simulink model "PubIfDecisionTOS_MDL"  (R2020b)
settings: configuration reference "DspaceConfig" (kept outside this file)
PostLoadFcn:
  | if any(exist('dsrtsu_mdlpostloadfcn', 'file') ~= 0), dsrtsu_mdlpostloadfcn('Execute', bdroot); end
InitFcn:
  | , if any(exist('dsmpb_private', 'file') ~= 0), dsmpb_private('dsmpb_mdlclblib', 'Init', bdroot); end,
undefined symbols (not defined in the file or in its folder): C_TOS_ACCEgoRAxletoFbumplength_m, C_TOS_ACCTargetFront_Flag, C_TOS_AEBJAPedObjDxThre_Val, C_TOS_AEBJAPedObjDyThre_Val, C_TOS_AEBJATargetSize_Val, C_TOS_AEBJAVehObjDxThre_Val, C_TOS_AEBJAVehObjDyThre_Val, C_TOS_AEBJuncPedTargetSize_Val, C_TOS_AEBLatObjDxThre_Val, C_TOS_AEBLatPedDyThre_Val, C_TOS_AEBLatTargetSize_Val, C_TOS_AEBLongTargetInEgoFront_Flag, C_TOS_axAbsGround_Parameter, C_TOS_CameraConfirmedFlag, C_TOS_CNsubjWidth, C_TOS_CurrentLaneCoreMinWidth_Val, C_TOS_CutInProb_Val_Zero, C_TOS_CutOutProb_Val_Zero, C_TOS_D2R_Val, C_TOS_DefaultValueObjectToCenterLine_dy, C_TOS_EgoCarWidth_Val, C_TOS_EgoDxRefPoint_m, C_TOS_EgoRAxletoFbumplength_m, C_TOS_HalfWidthVehicle_Con, C_TOS_HWA_CurrentLaneFlag, C_TOS_HWA_LeftLaneFlag, C_TOS_HWA_MovingDir_Vaild, C_TOS_HWA_MovState_Vaild, C_TOS_HWA_RightLaneFlag, C_TOS_LaneLineCourseErrorFront, C_TOS_LaneLineCourseErrorRear, C_TOS_MotorbikeDefaultWidth_m, C_TOS_NumberOfEffectiveTargets, C_TOS_Obj_Age_Val, C_TOS_Objdx_Constraint_Val, C_TOS_ObjectDefaultWidth_m, C_TOS_ObjInCurrentLane_Val, C_TOS_ObjInCurrentLaneValid, C_TOS_ObjInLeftLaneValid, C_TOS_ObjInRightLaneValid, C_TOS_ObjNotInCurrentLane_Val, C_TOS_ObjNotREElementType, C_TOS_ObjPredictDis_dy_ConstantVal_Zeros, C_TOS_ObjToCenterLine_ConstantVal_Zeros, C_TOS_OFMObjIDInvilad_Val, C_TOS_PIL_LatDisCons_Val_zero, C_TOS_PIL_ObjectCutInFlag_b, C_TOS_PIL_ObjectCutOutFlag_b, C_TOS_PIL_ObjLaneProb_al_Val, C_TOS_PP_ObjFusType_FC_Confirm_b, C_TOS_PP_ObjFusType_FC_FR_Confirm_b, C_TOS_PP_ObjFusType_FR_Confirm_b, C_TOS_RE_80BoolDefault_Val, C_TOS_RE_80Single181Default_Val, C_TOS_RE_80Single255Default_Val, C_TOS_RE_80Uint8Default_Val, C_TOS_RE_D2R, C_TOS_RE_D_180_Val, C_TOS_RE_InvalidObjectID_Val, C_TOS_RE_InvalidTargetChainDir_Val ... (+142)
libraries: simulink x1650, TOS_LIB x361, canfdmsglib x14
(part 39 of 69)

== system PubIfDecisionTOS_MDL/TOS_20201112/TOS_2012080320/TOS/AEB/TOS_AEBLong/AEBLong_Confirm/AEBLong/AEBLong_TrgConfirm/AEBLongTrgJudg ==
  ObjectID : Inport
  Object_DX : Inport  Port=2
  Object_ObstacleProb : Inport  Port=3
  Object_ExistProb : Inport  Port=4
  Object_Fus_Type : Inport  Port=5
  object_MovingState : Inport  Port=6
  Object_HeadingAngle : Inport  Port=7
  Object_Type : Inport  Port=8
  VIE_EgoVelocity : Inport  Port=9
  PIL_LeftLaneProb : Inport  Port=10
  PIL_CurrentLaneProb : Inport  Port=11
  PIL_RightLaneProb : Inport  Port=12
  PP_MovingStateSignalProcessing : Inport  Port=13
  PP_ObjMovingDirSignalProcessing : Inport  Port=14
  PP_ObjectToCenterLine_dy : Inport  Port=15
  PP_CurrentLaneWidth : Inport  Port=16
  TLJ_TargetInCLValidityflg : Inport  Port=17
  Object_DY : Inport  Port=18
  PP_ObjFusType_FC_FR_Confirm : Inport  Port=19
  PP_ObjFusType_FR_Confirm : Inport  Port=20
  PP_ObjFusType_FC_Confirm : Inport  Port=21
  Object_VX : Inport  Port=22
  Object_VY : Inport  Port=23
  PIL_OverlapRatio : Inport  Port=24
  AEBLong_Target_ID_K1 : Inport  Port=25
  AEBLong_Target_ID_K2 : Inport  Port=26
  AEBLong_Target_MovState_K1 : Inport  Port=27
  AEBLong_Target_MovState_K2 : Inport  Port=28
  SteerWheelAng : Inport  Port=29
  SteerWheelSpd : Inport  Port=30
  AEBLong_OverlapRatio : Subsystem
  Bus Creator : BusCreator  Inputs=30
  Bus Selector : BusSelector  OutputSignals=object_MovingState,PP_ObjFusType_FC_FR_Confirm,PP_ObjFusType_FR_Confirm,AEBLong_Target_ID_K1,AEBLong_Target_ID_K2,AEBLong_Target_MovState_K1,AEBLong_Target_MovState_K2,ObjectID
  Bus Selector1 : BusSelector  OutputSignals=object_MovingState,PP_ObjMovingDirSignalProcessing,Object_HeadingAngle,Object_VX,Object_VY,VIE_EgoVelocity,SteerWheelAng,AEBLong_Target_ID_K1,AEBLong_Target_ID_K2,AEBLong_Target_MovState_K1,AEBLong_Target_MovState_K2,ObjectID
  Bus Selector2 : BusSelector  OutputSignals=Object_DX,TLJ_TargetInCLValidityflg
  Bus Selector3 : BusSelector  OutputSignals=VIE_EgoVelocity,Object_DX
  Bus Selector4 : BusSelector  OutputSignals=Object_ExistProb
  Bus Selector5 : BusSelector  OutputSignals=PP_ObjFusType_FR_Confirm,object_MovingState,Object_DX,PP_ObjectToCenterLine_dy,Object_Type
  Bus Selector6 : BusSelector  OutputSignals=Object_DY,Object_DX,Object_Type
  Bus Selector7 : BusSelector  OutputSignals=Object_ObstacleProb,AEBLong_Target_ID_K1,ObjectID
  Bus Selector8 : BusSelector  OutputSignals=SteerWheelAng,SteerWheelSpd
  Bus Selector9 : BusSelector  OutputSignals=PIL_OverlapRatio
  Constant : Constant  OutDataTypeStr=boolean
  Constant2 : Constant  OutDataTypeStr=boolean
  Logical Operator : Logic  Inputs=10  AllPortsSameDT=off  OutDataTypeStr=boolean
  TOS_AEBLong_Dy : Subsystem
  TOS_AEBLong_ObjFusType : Subsystem
  TOS_AEBLong_ObstacleProb : Subsystem
  TOS_AEBLong_SteerWheelAngConfirm : Subsystem
  TOS_AEBLong_TargetDis : Subsystem
  TOS_AEBLong_TargetExistProb : Subsystem
  TOS_AEBLong_TargetInEgoFront : Subsystem
  TOS_AEBLong_TargetMovingDir : Subsystem
  TOS_AEB_Stockade : Subsystem
  Terminator : Terminator
  Terminator1 : Terminator
  TOS_AEBLong_TargetConditionJudge : Outport
  TOS_AEBLong_TargetDis_ObserVale : Outport  Port=2
  TOS_AEBLong_ObstacleProb_ObserVale : Outport  Port=3
  TOS_AEBLong_TargetExistProb_ObserVale : Outport  Port=4
  TOS_AEBLong_ObjFusType_ObserVale : Outport  Port=5
  TOS_AEBLong_TargetInEgoFront_ObserVale : Outport  Port=6
  TOS_AEBLong_TargetMovingDir_ObserVale : Outport  Port=7
  TOS_AEB_Stockade_ObserVale : Outport  Port=8
  TOS_AEBLong_TargetDy_ObserVale : Outport  Port=9
  TOS_AEBLong_SteerWheelAngConfirm_ObserVale : Outport  Port=10
  TOS_AEBLong_OverlapRatio_ObserVale : Outport  Port=11
  wires:
  TOS_AEBLong_ObjFusType/1(TOS_AEBLongAEBLongObjFusType) -> [TOS_AEBLong_ObjFusType_ObserVale], Logical Operator/4  "TOS_AEBLong_ObjFusType"
  TOS_AEBLong_ObstacleProb/1(TOS_AEBLongObstacleProbFlag) -> Logical Operator/2, [TOS_AEBLong_ObstacleProb_ObserVale]  "TOS_AEBLong_ObstacleProb"
  TOS_AEBLong_TargetExistProb/1(TOS_AEBLongTargetExistProbFlag) -> [TOS_AEBLong_TargetExistProb_ObserVale], Logical Operator/3  "TOS_AEBLong_TargetExistProb"
  Constant2/1 -> [TOS_AEB_Stockade_ObserVale], Logical Operator/7  "TOS_AEB_Stockade"
  TOS_AEBLong_TargetMovingDir/1(TOS_AEBLongMovingDirFlg) -> [TOS_AEBLong_TargetMovingDir_ObserVale], Logical Operator/6  "TOS_AEBLong_TargetMovingDir"
  TOS_AEBLong_TargetInEgoFront/1(TOS_TargetInEgoFrontflg) -> [TOS_AEBLong_TargetInEgoFront_ObserVale], Logical Operator/5  "TOS_AEBLong_TargetInEgoFront"
  TOS_AEBLong_TargetDis/1(TOS_TargetDxThreflg) -> Logical Operator/1, [TOS_AEBLong_TargetDis_ObserVale]  "TOS_AEBLong_TargetDis"
  Object_Fus_Type/1 -> Bus Creator/5  "Object_Fus_Type"
  PP_ObjMovingDirSignalProcessing/1 -> Bus Creator/14  "PP_ObjMovingDirSignalProcessing"
  PP_ObjectToCenterLine_dy/1 -> Bus Creator/15  "PP_ObjectToCenterLine_dy"
  VIE_EgoVelocity/1 -> Bus Creator/9  "VIE_EgoVelocity"
  Object_ExistProb/1 -> Bus Creator/4  "Object_ExistProb"
  PIL_CurrentLaneProb/1 -> Bus Creator/11  "PIL_CurrentLaneProb"
  PP_MovingStateSignalProcessing/1 -> Bus Creator/13  "PP_MovingStateSignalProcessing"
  PIL_RightLaneProb/1 -> Bus Creator/12  "PIL_RightLaneProb"
  PIL_LeftLaneProb/1 -> Bus Creator/10  "PIL_LeftLaneProb"
  Object_ObstacleProb/1 -> Bus Creator/3  "Object_ObstacleProb"
  Object_DX/1 -> Bus Creator/2  "Object_DX"
  PP_CurrentLaneWidth/1 -> Bus Creator/16  "PP_CurrentLaneWidth"
  Bus Selector1/2 -> TOS_AEBLong_TargetMovingDir/2(PP_ObjMovingDirSignalProcessing)  "<PP_ObjMovingDirSignalProcessing>"
  Bus Selector2/1 -> TOS_AEBLong_TargetInEgoFront/1(Object_Dx)  "<Object_DX>"
  Bus Selector7/1 -> TOS_AEBLong_ObstacleProb/1(Object_ObstacleProb)  "<Object_ObstacleProb>"
  Bus Selector3/1 -> TOS_AEBLong_TargetDis/1(VIE_EgoVelocity)  "<VIE_EgoVelocity>"
  Bus Selector4/1 -> TOS_AEBLong_TargetExistProb/1(Object_ExistProb)  "<Object_ExistProb>"
  Bus Selector3/2 -> TOS_AEBLong_TargetDis/2(Object_Dx)  "<Object_DX>"
  TLJ_TargetInCLValidityflg/1 -> Bus Creator/17  "TLJ_TargetInCLValidityflg"
  Bus Selector2/2 -> TOS_AEBLong_TargetInEgoFront/2(TLJ_TargetInCLValidityflg)  "<TLJ_TargetInCLValidityflg>"
  Bus Selector5/1 -> TOS_AEB_Stockade/1(PP_ObjFusType_FR_Confirm)  "<PP_ObjFusType_FR_Confirm>"
  Bus Selector5/2 -> TOS_AEB_Stockade/2(object_MovingState)  "<object_MovingState>"
  Bus Selector5/3 -> TOS_AEB_Stockade/3(Object_DX)  "<Object_DX>"
  Bus Selector5/4 -> TOS_AEB_Stockade/4(ObjectToCenterLine_dy)  "<PP_ObjectToCenterLine_dy>"
  [TOS_AEBLong_TargetDis_ObserVale] -> TOS_AEBLong_TargetDis_ObserVale/1
  [TOS_AEBLong_ObstacleProb_ObserVale] -> TOS_AEBLong_ObstacleProb_ObserVale/1
  [TOS_AEBLong_ObjFusType_ObserVale] -> TOS_AEBLong_ObjFusType_ObserVale/1
  [TOS_AEBLong_TargetExistProb_ObserVale] -> TOS_AEBLong_TargetExistProb_ObserVale/1
  [TOS_AEBLong_TargetInEgoFront_ObserVale] -> TOS_AEBLong_TargetInEgoFront_ObserVale/1
  [TOS_AEBLong_TargetMovingDir_ObserVale] -> TOS_AEBLong_TargetMovingDir_ObserVale/1
  [TOS_AEB_Stockade_ObserVale] -> TOS_AEB_Stockade_ObserVale/1
  TOS_AEBLong_Dy/1(TOS_AEBLongDy) -> [TOS_AEBLong_TargetDy_ObserVale], Logical Operator/8  "TOS_AEBLongDyFlag"
  Object_DY/1 -> Bus Creator/18  "Object_DY"
  [TOS_AEBLong_TargetDy_ObserVale] -> TOS_AEBLong_TargetDy_ObserVale/1
  object_MovingState/1 -> Bus Creator/6  "object_MovingState"
  Bus Selector/1 -> TOS_AEBLong_ObjFusType/1(object_MovingState)  "<object_MovingState>"
  Object_HeadingAngle/1 -> Bus Creator/7  "Object_HeadingAngle"
  Bus Selector1/3 -> TOS_AEBLong_TargetMovingDir/3(Object_HeadingAngle)  "<Object_HeadingAngle>"
  Object_Type/1 -> Bus Creator/8  "Object_Type"
  Bus Selector5/5 -> TOS_AEB_Stockade/5(Object_Type)  "<Object_Type>"
  Bus Selector1/1 -> TOS_AEBLong_TargetMovingDir/1(object_MovingState)  "<object_MovingState>"
  SteerWheelSpd/1 -> Bus Creator/20  "SteerWheelSpd"
  SteerWheelAng/1 -> Bus Creator/19  "SteerWheelAng"
  Bus Selector8/1 -> TOS_AEBLong_SteerWheelAngConfirm/1(SteerWheelAng)  "<SteerWheelAng>"
  Bus Selector8/2 -> TOS_AEBLong_SteerWheelAngConfirm/2(SteerWheelSpd)  "<SteerWheelSpd>"
  [TOS_AEBLong_SteerWheelAngConfirm_ObserVale] -> TOS_AEBLong_SteerWheelAngConfirm_ObserVale/1
  TOS_AEBLong_SteerWheelAngConfirm/1(TOS_AEBLong_SteerWheelAngConfirm) -> Logical Operator/9, [TOS_AEBLong_SteerWheelAngConfirm_ObserVale]  "TOS_AEBLong_SteerWheelAngConfirm"
  ObjectID/1 -> Bus Creator/1  "ObjectID"
  Logical Operator/1 -> TOS_AEBLong_TargetConditionJudge/1
  PP_ObjFusType_FC_FR_Confirm/1 -> Bus Creator/21  "PP_ObjFusType_FC_FR_Confirm"
  PP_ObjFusType_FR_Confirm/1 -> Bus Creator/22  "PP_ObjFusType_FR_Confirm"
  PP_ObjFusType_FC_Confirm/1 -> Bus Creator/23  "PP_ObjFusType_FC_Confirm"
  Bus Selector/2 -> TOS_AEBLong_ObjFusType/2(PP_ObjFusType_FC_FR_Confirm)  "<PP_ObjFusType_FC_FR_Confirm>"
  Bus Selector/3 -> TOS_AEBLong_ObjFusType/3(PP_ObjFusType_FR_Confirm)  "<PP_ObjFusType_FR_Confirm>"
  Bus Creator/1 -> Bus Selector6/1, Bus Selector9/1, Bus Selector8/1, Bus Selector5/1, Bus Selector1/1, Bus Selector2/1, Bus Selector/1, Bus Selector4/1, Bus Selector7/1, Bus Selector3/1
  Bus Selector6/2 -> TOS_AEBLong_Dy/2(Object_DX)  "<Object_DX>"
  Bus Selector6/1 -> TOS_AEBLong_Dy/1(Object_DY)  "<Object_DY>"
  Bus Selector6/3 -> TOS_AEBLong_Dy/3(<Object_Type>)  "<Object_Type>"
  Object_VY/1 -> Bus Creator/25  "Object_VY"
  Object_VX/1 -> Bus Creator/24  "Object_VX"
  Bus Selector1/4 -> TOS_AEBLong_TargetMovingDir/4(Object_VX)  "<Object_VX>"
  Bus Selector1/5 -> TOS_AEBLong_TargetMovingDir/5(Object_VY)  "<Object_VY>"
  Bus Selector1/6 -> TOS_AEBLong_TargetMovingDir/6(VIE_EgoVelocity)  "<VIE_EgoVelocity>"
  Bus Selector1/7 -> TOS_AEBLong_TargetMovingDir/7(SteerWheelAngle)  "<SteerWheelAng>"
  PIL_OverlapRatio/1 -> Bus Creator/26  "PIL_OverlapRatio"
  Bus Selector9/1 -> AEBLong_OverlapRatio/1(PIL_OverlapRatio)  "<PIL_OverlapRatio>"
  Constant/1 -> [TOS_AEBLong_OverlapRatio_ObserVale], Logical Operator/10
  [TOS_AEBLong_OverlapRatio_ObserVale] -> TOS_AEBLong_OverlapRatio_ObserVale/1
  AEBLong_OverlapRatio/1(AEBLong_OverlapRatioFlag) -> Terminator/1
  TOS_AEB_Stockade/1(TOS_AEB_Stockade) -> Terminator1/1
  AEBLong_Target_ID_K1/1 -> Bus Creator/27  "AEBLong_Target_ID_K1"
  AEBLong_Target_ID_K2/1 -> Bus Creator/28  "AEBLong_Target_ID_K2"
  AEBLong_Target_MovState_K1/1 -> Bus Creator/29  "AEBLong_Target_MovState_K1"
  AEBLong_Target_MovState_K2/1 -> Bus Creator/30  "AEBLong_Target_MovState_K2"
  Bus Selector/4 -> TOS_AEBLong_ObjFusType/4(AEBLong_Target_ID_K1)  "<AEBLong_Target_ID_K1>"
  Bus Selector/5 -> TOS_AEBLong_ObjFusType/5(AEBLong_Target_ID_K2)  "<AEBLong_Target_ID_K2>"
  Bus Selector/6 -> TOS_AEBLong_ObjFusType/6(AEBLong_Target_MovState_K1)  "<AEBLong_Target_MovState_K1>"
  Bus Selector/7 -> TOS_AEBLong_ObjFusType/7(AEBLong_Target_MovState_K2)  "<AEBLong_Target_MovState_K2>"
  Bus Selector/8 -> TOS_AEBLong_ObjFusType/8(ObjectID)  "<ObjectID>"
  Bus Selector7/2 -> TOS_AEBLong_ObstacleProb/2(AEBLong_Target_ID_K1)  "<AEBLong_Target_ID_K1>"
  Bus Selector7/3 -> TOS_AEBLong_ObstacleProb/3(ObjectID)  "<ObjectID>"
  Bus Selector1/8 -> TOS_AEBLong_TargetMovingDir/8(AEBLong_Target_ID_K1)  "<AEBLong_Target_ID_K1>"
  Bus Selector1/9 -> TOS_AEBLong_TargetMovingDir/9(AEBLong_Target_ID_K2)  "<AEBLong_Target_ID_K2>"
  Bus Selector1/10 -> TOS_AEBLong_TargetMovingDir/10(AEBLong_Target_MovState_K1)  "<AEBLong_Target_MovState_K1>"
  Bus Selector1/11 -> TOS_AEBLong_TargetMovingDir/11(AEBLong_Target_MovState_K2)  "<AEBLong_Target_MovState_K2>"
  Bus Selector1/12 -> TOS_AEBLong_TargetMovingDir/12(ObjectID)  "<ObjectID>"

== system PubIfDecisionTOS_MDL/TOS_20201112/TOS_2012080320/TOS/AEB/TOS_AEBLong/AEBLong_Confirm/AEBLong/AEBLong_TrgConfirm/Subsystem ==
  Dx1stNearestObjIndex : Inport
  Object_ID : Inport  Port=2
  Object_DX : Inport  Port=3
  Object_ObstacleProb : Inport  Port=4
  Object_ExistProb : Inport  Port=5
  Object_Fus_Type : Inport  Port=6
  object_MovingState : Inport  Port=7
  Object_HeadingAngle : Inport  Port=8
  Object_Type : Inport  Port=9
  VIE_EgoVelocity : Inport  Port=10
  PIL_LeftLaneProb : Inport  Port=11
  PIL_CurrentLaneProb : Inport  Port=12
  PIL_RightLaneProb : Inport  Port=13
  PP_MovingStateSignalProcessing : Inport  Port=14
  PP_ObjMovingDirSignalProcessing : Inport  Port=15
  PP_ObjectToCenterLine_dy : Inport  Port=16
  TLJ_TargetInCLValidityflg : Inport  Port=17
  PP_CurrentLaneWidth : Inport  Port=18
  Object_DY : Inport  Port=19
  PP_ObjFusType_FC_FR_Confirm : Inport  Port=20
  PP_ObjFusType_FR_Confirm : Inport  Port=21
  PP_ObjFusType_FC_Confirm : Inport  Port=22
  Object_VX : Inport  Port=23
  Object_VY : Inport  Port=24
  PIL_OverlapRatio : Inport  Port=25
  AEBLong_Target_ID_K1 : Inport  Port=26
  AEBLong_Target_ID_K2 : Inport  Port=27
  AEBLong_Target_MovState_K1 : Inport  Port=28
  AEBLong_Target_MovState_K2 : Inport  Port=29
  Selector{,1..21} (22 alike) : Selector  InputPortWidth=80  IndexOptions=Index vector (port)  Indices=[1 3]  OutputSizes=1
  ObjectID : Outport
  ObjectDX : Outport  Port=2
  ObjectObstacleProb : Outport  Port=3
  ObjectExistProb : Outport  Port=4
  ObjectFus_Type : Outport  Port=5
  objectMovingState : Outport  Port=6
  ObjectHeadingAngle : Outport  Port=7
  ObjectType : Outport  Port=8
  VIEEgoVelocity : Outport  Port=9
  PILLeftLaneProb : Outport  Port=10
  PILCurrentLaneProb : Outport  Port=11
  PILRightLaneProb : Outport  Port=12
  PPMovingStateSignalProcessing : Outport  Port=13
  PPObjMovingDirSignalProcessing : Outport  Port=14
  PPObjectToCenterLine_dy : Outport  Port=15
  PPCurrentLaneWidth : Outport  Port=16
  TLJTargetInCLValidityflg : Outport  Port=17
  ObjectDY : Outport  Port=18
  PP_ObjFusType_FC_FR_Confirm_ : Outport  Port=19
  PP_ObjFusType_FR_Confirm_ : Outport  Port=20
  PP_ObjFusType_FC_Confirm_ : Outport  Port=21
  ObjectVX : Outport  Port=22
  ObjectVY : Outport  Port=23
  PILOverlapRatio : Outport  Port=24
  AEBLongTarget_ID_K2 : Outport  Port=25
  AEBLongTarget_ID_K1 : Outport  Port=26
  AEBLongTarget_MovState_K2 : Outport  Port=27
  AEBLongTarget_MovState_K1 : Outport  Port=28
  wires:
  Object_ID/1 -> Selector/1
  Object_ObstacleProb/1 -> Selector2/1
  Object_DX/1 -> Selector1/1
  Selector/1 -> ObjectID/1  "Object_ID"
  Object_ExistProb/1 -> Selector3/1
  Object_DY/1 -> Selector16/1
  Object_Fus_Type/1 -> Selector4/1
  object_MovingState/1 -> Selector5/1
  Object_HeadingAngle/1 -> Selector6/1
  Object_Type/1 -> Selector7/1
  PIL_LeftLaneProb/1 -> Selector8/1
  PIL_CurrentLaneProb/1 -> Selector9/1
  PIL_RightLaneProb/1 -> Selector10/1
  PP_MovingStateSignalProcessing/1 -> Selector11/1
  PP_ObjMovingDirSignalProcessing/1 -> Selector12/1
  PP_ObjectToCenterLine_dy/1 -> Selector13/1
  TLJ_TargetInCLValidityflg/1 -> Selector15/1
  Selector1/1 -> ObjectDX/1  "Object_DX"
  Selector2/1 -> ObjectObstacleProb/1  "Object_ObstacleProb"
  Selector3/1 -> ObjectExistProb/1  "Object_ExistProb"
  Selector4/1 -> ObjectFus_Type/1  "Object_Fus_Type"
  Selector5/1 -> objectMovingState/1  "object_MovingState"
  Selector6/1 -> ObjectHeadingAngle/1  "Object_HeadingAngle"
  Selector7/1 -> ObjectType/1  "Object_Type"
  VIE_EgoVelocity/1 -> VIEEgoVelocity/1  "VIE_EgoVelocity"
  Selector8/1 -> PILLeftLaneProb/1  "PIL_LeftLaneProb"
  Selector9/1 -> PILCurrentLaneProb/1  "PIL_CurrentLaneProb"
  Selector10/1 -> PILRightLaneProb/1  "PIL_RightLaneProb"
  Selector11/1 -> PPMovingStateSignalProcessing/1  "PP_MovingStateSignalProcessing"
  Selector12/1 -> PPObjMovingDirSignalProcessing/1  "PP_ObjMovingDirSignalProcessing"
  Selector13/1 -> PPObjectToCenterLine_dy/1  "PP_ObjectToCenterLine_dy"
  PP_CurrentLaneWidth/1 -> PPCurrentLaneWidth/1  "PP_CurrentLaneWidth"
  Selector15/1 -> TLJTargetInCLValidityflg/1  "TLJ_TargetInCLValidityflg"
  Selector16/1 -> ObjectDY/1  "Object_DY"
  PP_ObjFusType_FC_FR_Confirm/1 -> Selector14/1
  PP_ObjFusType_FR_Confirm/1 -> Selector17/1
  PP_ObjFusType_FC_Confirm/1 -> Selector18/1
  Selector18/1 -> PP_ObjFusType_FC_Confirm_/1
  Selector17/1 -> PP_ObjFusType_FR_Confirm_/1
  Selector14/1 -> PP_ObjFusType_FC_FR_Confirm_/1
  Selector19/1 -> ObjectVX/1
  Object_VX/1 -> Selector19/1
  Selector20/1 -> ObjectVY/1
  Object_VY/1 -> Selector20/1
  PIL_OverlapRatio/1 -> Selector21/1
  Dx1stNearestObjIndex/1 -> Selector1/2, Selector2/2, Selector3/2, Selector4/2, Selector5/2, Selector6/2, Selector7/2, Selector8/2, Selector9/2, Selector10/2, Selector11/2, Selector12/2, Selector13/2, Selector21/2, Selector20/2, Selector19/2, Selector18/2, Selector17/2, Selector14/2, Selector16/2, Selector15/2, Selector/2
  Selector21/1 -> PILOverlapRatio/1
  AEBLong_Target_ID_K1/1 -> AEBLongTarget_ID_K1/1  "AEBLong_Target_ID_K1"
  AEBLong_Target_ID_K2/1 -> AEBLongTarget_ID_K2/1  "AEBLong_Target_ID_K2"
  AEBLong_Target_MovState_K1/1 -> AEBLongTarget_MovState_K1/1
  AEBLong_Target_MovState_K2/1 -> AEBLongTarget_MovState_K2/1

== system PubIfDecisionTOS_MDL/TOS_20201112/TOS_2012080320/TOS/AEB/TOS_AEBLong/AEBLong_Target_PreJudge/AEBLONG_Target_PreFilt/AEBLONG_TargetPreCondJudge/AEBLONGTarget_Fence ==
  FR_Confirm : Inport
  Obj_MovingState : Inport  Port=2
  Object_ObstacleProb : Inport  Port=3
  Object_DY : Inport  Port=4
  Chart : Stateflow chart  TreatAsAtomicUnit=on
  Data Type Conversion1 : DataTypeConversion  OutDataTypeStr=Enum: OFM_OBJ_MOVINGSTATE_E
  TOS_AEBLONG_Target_FenceFlag : Outport
  wires:
  Chart/1(ObjectisFence_Flag) -> TOS_AEBLONG_Target_FenceFlag/1
  Object_DY/1 -> Chart/4(Object_DY)
  FR_Confirm/1 -> Chart/1(FR_Confirm)
  Obj_MovingState/1 -> Data Type Conversion1/1
  Object_ObstacleProb/1 -> Chart/3(Object_ObstacleProb)
  Data Type Conversion1/1 -> Chart/2(Obj_MovingState)

== system PubIfDecisionTOS_MDL/TOS_20201112/TOS_2012080320/TOS/AEB/TOS_AEBLong/AEBLong_Target_PreJudge/AEBLONG_Target_PreFilt/AEBLONG_TargetPreCondJudge/AEBLONGTarget_FusionType ==
  PP_ObjFusType_FC_FR_Confirm : Inport
  PP_ObjFusType_FR_Confirm : Inport  Port=2
  Compare To Constant5 : simulink/Logic and Bit Operations/Compare To Constant  relop===  const=C_TOS_PP_ObjFusType_FC_FR_Confirm_b  OutDataTypeStr=boolean
      settings: AttributesFormatString=C_TOS_PP_ObjFusType_FC_FR_Confirm_b = 1
  Compare To Constant6 : simulink/Logic and Bit Operations/Compare To Constant  relop===  const=C_TOS_PP_ObjFusType_FR_Confirm_b  OutDataTypeStr=boolean
      settings: AttributesFormatString=C_TOS_PP_ObjFusType_FR_Confirm_b = 1
  Logical Operator : Logic  Operator=OR  AllPortsSameDT=off  OutDataTypeStr=boolean
  TOS_AEBLONG_Target_FusionTypeFlag : Outport
  wires:
  Logical Operator/1 -> TOS_AEBLONG_Target_FusionTypeFlag/1
  Compare To Constant6/1 -> Logical Operator/2
  PP_ObjFusType_FC_FR_Confirm/1 -> Compare To Constant5/1
  PP_ObjFusType_FR_Confirm/1 -> Compare To Constant6/1
  Compare To Constant5/1 -> Logical Operator/1

== system PubIfDecisionTOS_MDL/TOS_20201112/TOS_2012080320/TOS/AEB/TOS_AEBLong/AEBLong_Target_PreJudge/AEBLONG_Target_PreFilt/AEBLONG_TargetPreCondJudge/AEBLONGTarget_PassedbyTarget ==
  note: 目标分裂处理
  FR_Confirm : Inport
  Obj_MovingState : Inport  Port=2
  Obj_Dx : Inport  Port=3
  AEBLONG_TargetP0_ID_K1 : Inport  Port=4
  AEBLONG_TargetP0_Dx_K1 : Inport  Port=5
  Object_ID : Inport  Port=6
  Add : Sum
  Compare To Constant : simulink/Logic and Bit Operations/Compare To Constant  relop=~=  const=C_TOS_OFMObjIDInvilad_Val  OutDataTypeStr=boolean
      settings: AttributesFormatString=C_TOS_OFMObjIDInvilad_Val = 0
  Compare To Constant1 : simulink/Logic and Bit Operations/Compare To Constant  relop===  const=C_TOS_PP_ObjFusType_FR_Confirm_b  OutDataTypeStr=boolean
      settings: AttributesFormatString=C_TOS_PP_ObjFusType_FC_Confirm_b = 1
  Compare To Constant2 : simulink/Logic and Bit Operations/Compare To Constant  relop===  const=OFM_OBJ_MOVINGSTATE_E.UNKNOWN  OutDataTypeStr=boolean
      settings: AttributesFormatString=OFM_OBJ_MOVINGSTATE_E.MOVING = 2
  Compare To Constant3 : simulink/Logic and Bit Operations/Compare To Constant  relop===  const=OFM_OBJ_MOVINGSTATE_E.INVALID  OutDataTypeStr=boolean
      settings: AttributesFormatString=OFM_OBJ_MOVINGSTATE_E.MOVING = 2
  Compare To Constant4 : simulink/Logic and Bit Operations/Compare To Constant  relop===  const=OFM_OBJ_MOVINGSTATE_E.STATIONARY  OutDataTypeStr=boolean
      settings: AttributesFormatString=OFM_OBJ_MOVINGSTATE_E.MOVING = 2
  Constant : Constant  OutDataTypeStr=single
  Constant1 : Constant  Value=0  OutDataTypeStr=boolean
  Constant2 : Constant  Value=0  OutDataTypeStr=boolean
  Data Type Conversion1 : DataTypeConversion  OutDataTypeStr=Enum: OFM_OBJ_MOVINGSTATE_E
  Logical Operator : Logic  Operator=OR  Inputs=3  AllPortsSameDT=off  OutDataTypeStr=boolean
  Logical Operator1 : Logic  AllPortsSameDT=off  OutDataTypeStr=boolean
  Logical Operator2 : Logic  AllPortsSameDT=off  OutDataTypeStr=boolean
  Relational Operator : RelationalOperator  Operator=<  OutDataTypeStr=boolean  RndMeth=Simplest
  Relational Operator1 : RelationalOperator  Operator=~=  OutDataTypeStr=boolean  RndMeth=Simplest
  Switch : Switch  Criteria=u2 ~= 0
  Switch1 : Switch  Criteria=u2 ~= 0
  TOS_AEBLONG_Target_PassedbyTarget_Flag : Outport
  wires:
  Switch/1 -> TOS_AEBLONG_Target_PassedbyTarget_Flag/1
  Compare To Constant3/1 -> Logical Operator/1
  Compare To Constant/1 -> Logical Operator2/1
  Constant/1 -> Add/2
  Obj_MovingState/1 -> Data Type Conversion1/1
  Obj_Dx/1 -> Relational Operator/1
  Relational Operator/1 -> Switch1/1
  Compare To Constant1/1 -> Logical Operator1/1
  Compare To Constant2/1 -> Logical Operator/2
  FR_Confirm/1 -> Compare To Constant1/1
  Logical Operator1/1 -> Switch1/2
  Switch1/1 -> Switch/1
  Add/1 -> Relational Operator/2
  Logical Operator/1 -> Logical Operator1/2
  Constant2/1 -> Switch/3
  AEBLONG_TargetP0_Dx_K1/1 -> Add/1
  Constant1/1 -> Switch1/3
  Compare To Constant4/1 -> Logical Operator/3
  AEBLONG_TargetP0_ID_K1/1 -> Relational Operator1/1, Compare To Constant/1
  Data Type Conversion1/1 -> Compare To Constant4/1, Compare To Constant2/1, Compare To Constant3/1
  Object_ID/1 -> Relational Operator1/2
  Relational Operator1/1 -> Logical Operator2/2
  Logical Operator2/1 -> Switch/2

== system PubIfDecisionTOS_MDL/TOS_20201112/TOS_2012080320/TOS/AEB/TOS_AEBLong/AEBLong_Target_PreJudge/AEBLONG_Target_PreFilt/AEBLONG_TargetPreCondJudge/REElementType ==
  PP_REElementType : Inport
  Compare To Constant1 : simulink/Logic and Bit Operations/Compare To Constant  relop===  const=C_TOS_ObjNotREElementType  OutDataTypeStr=boolean
      settings: AttributesFormatString=%<const> = 0
  TOS_AEBLONG_Target_REElementType : Outport
  wires:
  Compare To Constant1/1 -> TOS_AEBLONG_Target_REElementType/1
  PP_REElementType/1 -> Compare To Constant1/1

== system PubIfDecisionTOS_MDL/TOS_20201112/TOS_2012080320/TOS/LC_LCKie_ELK/TOS_HWA/CurrentLane/HWA_CurrentLane_Target/HWA_CLF_Target_1/HWA_CLF_Target ==
  HWA_CLF_Target_1_Index : Inport
  Object_Fus_Type : Inport  Port=2
  object_MovingState : Inport  Port=3
  PP_ObjMovingDirSignalProcessing : Inport  Port=4
  Object_HeadingAngle : Inport  Port=5
  Object_DX : Inport  Port=6
  TOS_TLJ_SameLaneConfirm_Flag : Inport  Port=7
  Object_Type : Inport  Port=8
  Object_ObstacleProb : Inport  Port=9
  Object_DY : Inport  Port=10
  PP_ObjFusType_FC_FR_Confirm : Inport  Port=11
  PP_ObjFusType_FR_Confirm : Inport  Port=12
  PP_ObjFusType_FC_Confirm : Inport  Port=13
  Object_VX : Inport  Port=14
  Object_VY : Inport  Port=15
  VIE_EgoVelocity : Inport  Port=16
  SteerWheelAng : Inport  Port=17
  PIL_OverlapRatio : Inport  Port=18
  HWA_CLF_Target_ID_K1 : Inport  Port=19
  HWA_CLF_Target_Target_ID_K2 : Inport  Port=20
  HWA_CLF_Target_Target_MovState_K1 : Inport  Port=21
  HWA_CLF_Target_Target_MovState_K2 : Inport  Port=22
  ObjectID : Inport  Port=23
  LM_LR_Line04_dDisStart : Inport  Port=24
  LM_LR_Line04_dDisEnd : Inport  Port=25
  LM_LR_Line05_dDisStart : Inport  Port=26
  LM_LR_Line05_dDisEnd : Inport  Port=27
  LM_LR_Line06_dDisStart : Inport  Port=28
  LM_LR_Line06_dDisEnd : Inport  Port=29
  LM_LR_Line04_pC2 : Inport  Port=30
  LM_LR_Line05_pC2 : Inport  Port=31
  LM_LR_Line06_pC2 : Inport  Port=32
  LM_LR_Line04_fCamValid : Inport  Port=33
  LM_LR_Line05_fCamValid : Inport  Port=34
  LM_LR_Line06_fCamValid : Inport  Port=35
  LM_LR_Line04_pC0 : Inport  Port=36
  LM_RL_Line04_pC0 : Inport  Port=37
  Action Port : ActionPort  ActionPortLabel=else
  HWA_CLF_Target : Subsystem
  Selector{1..16} (16 alike) : Selector  InputPortWidth=80  IndexOptions=Index vector (port)  Indices=[1 3]  OutputSizes=1
  HWA_CLF_Target_1_TargeConfirm : Outport
  HWA_CLF_Target_FusionType_ObserVale : Outport  Port=2
  HWA_CLF_Target_TrgMovDir_ObserVale : Outport  Port=3
  HWA_CLF_Target_TargetDxConfirm_ObserVale : Outport  Port=4
  HWA_CLF_Target_ObjType_ObserVale : Outport  Port=5
  HWA_CLF_Target_ObstacleProb_ObserVale : Outport  Port=6
  HWA_CLF_Target_DyConfirm_ObserVale : Outport  Port=7
  HWA_CLF_Target_TrgMovDirFlag_1_ObserVale : Outport  Port=8
  HWA_CLF_Target_TrgMovDirFlag_2_ObserVale : Outport  Port=9
  HWA_CLF_Target_TrgMovDirFlag_3_ObserVale : Outport  Port=10
  HWA_CLF_Target_TrgMovDirFlag_4_ObserVale : Outport  Port=11
  HWA_CLF_Target_TrgMovDirFlag_5_ObserVale : Outport  Port=12
  HWA_CLF_Target_TrgMovDirFlag_6_ObserVale : Outport  Port=13
  HWA_CLF_Target_DyConfirm_1_ObserVale : Outport  Port=14
  HWA_CLF_Target_DyConfirm_2_ObserVale : Outport  Port=15
  HWA_CLF_Target_DyConfirm_3_ObserVale : Outport  Port=16
  HWA_CLF_Target_DyConfirm_4_OverlapRatio_ObserVale : Outport  Port=17
  HWA_CLF_Target_DyConfirm_5_OverlapConfirm_ObserVale : Outport  Port=18
  HWA_CLF_Target_DyConfirm_ALL_6_ObserVale : Outport  Port=19
  wires:
  LM_RL_Line04_pC0/1 -> HWA_CLF_Target/36(LM_RL_Line04_pC0)
  LM_LR_Line04_pC0/1 -> HWA_CLF_Target/35(LM_LR_Line04_pC0)
  HWA_CLF_Target/19(TOS_DyConfirm_ALL_6_ObserVale) -> HWA_CLF_Target_DyConfirm_ALL_6_ObserVale/1
  HWA_CLF_Target/18(TOS_DyConfirm_5_OverlapConfirm_ObserVale) -> HWA_CLF_Target_DyConfirm_5_OverlapConfirm_ObserVale/1
  HWA_CLF_Target/17(TOS_DyConfirm_4_OverlapRatio_ObserVale) -> HWA_CLF_Target_DyConfirm_4_OverlapRatio_ObserVale/1
  HWA_CLF_Target/16(TOS_DyConfirm_3_ObserVale) -> HWA_CLF_Target_DyConfirm_3_ObserVale/1
  HWA_CLF_Target/15(TOS_DyConfirm_2_ObserVale) -> HWA_CLF_Target_DyConfirm_2_ObserVale/1
  HWA_CLF_Target/14(TOS_DyConfirm_1_ObserVale) -> HWA_CLF_Target_DyConfirm_1_ObserVale/1
  HWA_CLF_Target/13(TOS_TrgMovDirFlag_6_ObserVale) -> HWA_CLF_Target_TrgMovDirFlag_6_ObserVale/1
  HWA_CLF_Target/12(TOS_TrgMovDirFlag_5_ObserVale) -> HWA_CLF_Target_TrgMovDirFlag_5_ObserVale/1
  HWA_CLF_Target/1(HWA_CLF_TargeConfirm) -> HWA_CLF_Target_1_TargeConfirm/1
  HWA_CLF_Target/11(TOS_TrgMovDirFlag_4_ObserVale) -> HWA_CLF_Target_TrgMovDirFlag_4_ObserVale/1
  HWA_CLF_Target/2(TOS_FusionType_ObserVale) -> HWA_CLF_Target_FusionType_ObserVale/1
  HWA_CLF_Target/10(TOS_TrgMovDirFlag_3_ObserVale) -> HWA_CLF_Target_TrgMovDirFlag_3_ObserVale/1
  HWA_CLF_Target/3(TOS_TrgMovDir_ObserVale) -> HWA_CLF_Target_TrgMovDir_ObserVale/1
  HWA_CLF_Target/9(TOS_TrgMovDirFlag_2_ObserVale) -> HWA_CLF_Target_TrgMovDirFlag_2_ObserVale/1
  HWA_CLF_Target/4(TOS_TargetDxConfirm_ObserVale) -> HWA_CLF_Target_TargetDxConfirm_ObserVale/1
  HWA_CLF_Target/8(TOS_TrgMovDirFlag_1_ObserVale) -> HWA_CLF_Target_TrgMovDirFlag_1_ObserVale/1
  HWA_CLF_Target/5(TOS_ObjType_ObserVale) -> HWA_CLF_Target_ObjType_ObserVale/1
  HWA_CLF_Target/7(TOS_DyConfirm_ObserVale) -> HWA_CLF_Target_DyConfirm_ObserVale/1
  HWA_CLF_Target/6(TOS_ObstacleProb_ObserVale) -> HWA_CLF_Target_ObstacleProb_ObserVale/1
  LM_LR_Line05_fCamValid/1 -> HWA_CLF_Target/33(LM_LR_Line05_fCamValid)
  LM_LR_Line04_fCamValid/1 -> HWA_CLF_Target/32(LM_LR_Line04_fCamValid)
  LM_LR_Line06_fCamValid/1 -> HWA_CLF_Target/34(LM_LR_Line06_fCamValid)
  LM_LR_Line05_pC2/1 -> HWA_CLF_Target/30(LM_LR_Line05_pC2)
  LM_LR_Line04_pC2/1 -> HWA_CLF_Target/29(LM_LR_Line04_pC2)
  LM_LR_Line06_dDisEnd/1 -> HWA_CLF_Target/28(LM_LR_Line06_dDisEnd)
  LM_LR_Line06_dDisStart/1 -> HWA_CLF_Target/27(LM_LR_Line06_dDisStart)
  LM_LR_Line05_dDisEnd/1 -> HWA_CLF_Target/26(LM_LR_Line05_dDisEnd)
  LM_LR_Line05_dDisStart/1 -> HWA_CLF_Target/25(LM_LR_Line05_dDisStart)
  LM_LR_Line04_dDisEnd/1 -> HWA_CLF_Target/24(LM_LR_Line04_dDisEnd)
  LM_LR_Line04_dDisStart/1 -> HWA_CLF_Target/23(LM_LR_Line04_dDisStart)
  LM_LR_Line06_pC2/1 -> HWA_CLF_Target/31(LM_LR_Line06_pC2)
  HWA_CLF_Target_1_Index/1 -> Selector16/2, Selector14/2, Selector11/2, Selector10/2, Selector9/2, Selector8/2, Selector7/2, Selector6/2, Selector5/2, Selector2/2, Selector4/2, Selector3/2, Selector15/2, Selector12/2, Selector13/2, Selector1/2
  Selector3/1 -> HWA_CLF_Target/22(ObjectID)
  Selector4/1 -> HWA_CLF_Target/17(PIL_OverlapRatio)
  Selector2/1 -> HWA_CLF_Target/14(Object_VY)
  Selector5/1 -> HWA_CLF_Target/13(Object_VX)
  Selector6/1 -> HWA_CLF_Target/12(PP_ObjFusType_FC_Confirm)
  Selector7/1 -> HWA_CLF_Target/11(PP_ObjFusType_FR_Confirm)
  Selector8/1 -> HWA_CLF_Target/10(PP_ObjFusType_FC_FR_Confirm)
  Selector9/1 -> HWA_CLF_Target/9(Object_DY)
  Selector10/1 -> HWA_CLF_Target/8(Object_ObstacleProb)
  Selector11/1 -> HWA_CLF_Target/7(Object_Type)
  Selector14/1 -> HWA_CLF_Target/6(TOS_TLJ_SameLaneConfirm_Flag)
  Selector15/1 -> HWA_CLF_Target/5(Object_DX)
  Selector16/1 -> HWA_CLF_Target/4(Object_HeadingAngle)
  Selector12/1 -> HWA_CLF_Target/3(PP_ObjMovingDirSignalProcessing)
  Selector13/1 -> HWA_CLF_Target/2(object_MovingState)
  Selector1/1 -> HWA_CLF_Target/1(Object_Fus_Type)
  ObjectID/1 -> Selector3/1
  HWA_CLF_Target_Target_MovState_K2/1 -> HWA_CLF_Target/21(HWA_CLF_Target_MovState_K2)
  HWA_CLF_Target_Target_MovState_K1/1 -> HWA_CLF_Target/20(HWA_CLF_Target_MovState_K1)
  HWA_CLF_Target_Target_ID_K2/1 -> HWA_CLF_Target/19(HWA_CLF_Target_ID_K2)
  HWA_CLF_Target_ID_K1/1 -> HWA_CLF_Target/18(HWA_CLF_Target_ID_K1)
  PIL_OverlapRatio/1 -> Selector4/1
  SteerWheelAng/1 -> HWA_CLF_Target/16(SteerWheelAng)
  VIE_EgoVelocity/1 -> HWA_CLF_Target/15(VIE_EgoVelocity)
  Object_VY/1 -> Selector2/1
  Object_VX/1 -> Selector5/1
  PP_ObjFusType_FC_Confirm/1 -> Selector6/1
  PP_ObjFusType_FR_Confirm/1 -> Selector7/1
  PP_ObjFusType_FC_FR_Confirm/1 -> Selector8/1
  Object_DY/1 -> Selector9/1
  Object_ObstacleProb/1 -> Selector10/1
  Object_Type/1 -> Selector11/1
  TOS_TLJ_SameLaneConfirm_Flag/1 -> Selector14/1
  Object_DX/1 -> Selector15/1
  Object_HeadingAngle/1 -> Selector16/1
  PP_ObjMovingDirSignalProcessing/1 -> Selector12/1
  object_MovingState/1 -> Selector13/1
  Object_Fus_Type/1 -> Selector1/1

== system PubIfDecisionTOS_MDL/TOS_20201112/TOS_2012080320/TOS/LC_LCKie_ELK/TOS_HWA/CurrentLane/HWA_CurrentLane_Target/HWA_CLF_Target_1/HWA_CLF_TargetDefault ==
  Action Port : ActionPort  ActionPortLabel=if(u1 ~= 0)
  Constant{1..19} (19 alike) : Constant  Value=0  OutDataTypeStr=boolean
  HWA_CLF_Target_2_TargeConfirm : Outport
  HWA_CLF_Target_FusionType_ObserVale : Outport  Port=2
  HWA_CLF_Target_TrgMovDir_ObserVale : Outport  Port=3
  HWA_CLF_Target_TargetDxConfirm_ObserVale : Outport  Port=4
  HWA_CLF_Target_ObjType_ObserVale : Outport  Port=5
  HWA_CLF_Target_ObstacleProb_ObserVale : Outport  Port=6
  HWA_CLF_Target_DyConfirm_ObserVale : Outport  Port=7
  HWA_CLF_Target_TrgMovDirFlag_1_ObserVale : Outport  Port=8
  HWA_CLF_Target_TrgMovDirFlag_2_ObserVale : Outport  Port=9
  HWA_CLF_Target_TrgMovDirFlag_3_ObserVale : Outport  Port=10
  HWA_CLF_Target_TrgMovDirFlag_4_ObserVale : Outport  Port=11
  HWA_CLF_Target_TrgMovDirFlag_5_ObserVale : Outport  Port=12
  HWA_CLF_Target_TrgMovDirFlag_6_ObserVale : Outport  Port=13
  HWA_CLF_Target_DyConfirm_1_ObserVale : Outport  Port=14
  HWA_CLF_Target_DyConfirm_2_ObserVale : Outport  Port=15
  HWA_CLF_Target_DyConfirm_3_ObserVale : Outport  Port=16
  HWA_CLF_Target_DyConfirm_4_OverlapRatio_ObserVale : Outport  Port=17
  HWA_CLF_Target_DyConfirm_5_OverlapConfirm_ObserVale : Outport  Port=18
  HWA_CLF_Target_DyConfirm_ALL_6_ObserVale : Outport  Port=19
  wires:
  Constant19/1 -> HWA_CLF_Target_DyConfirm_ALL_6_ObserVale/1
  Constant18/1 -> HWA_CLF_Target_DyConfirm_5_OverlapConfirm_ObserVale/1
  Constant17/1 -> HWA_CLF_Target_DyConfirm_1_ObserVale/1
  Constant16/1 -> HWA_CLF_Target_DyConfirm_4_OverlapRatio_ObserVale/1
  Constant15/1 -> HWA_CLF_Target_DyConfirm_3_ObserVale/1
  Constant14/1 -> HWA_CLF_Target_DyConfirm_2_ObserVale/1
  Constant13/1 -> HWA_CLF_Target_TrgMovDirFlag_6_ObserVale/1
  Constant12/1 -> HWA_CLF_Target_TrgMovDirFlag_5_ObserVale/1
  Constant11/1 -> HWA_CLF_Target_TrgMovDirFlag_4_ObserVale/1
  Constant10/1 -> HWA_CLF_Target_TrgMovDirFlag_3_ObserVale/1
  Constant9/1 -> HWA_CLF_Target_TrgMovDirFlag_2_ObserVale/1
  Constant8/1 -> HWA_CLF_Target_TrgMovDirFlag_1_ObserVale/1
  Constant7/1 -> HWA_CLF_Target_DyConfirm_ObserVale/1
  Constant6/1 -> HWA_CLF_Target_ObstacleProb_ObserVale/1
  Constant5/1 -> HWA_CLF_Target_ObjType_ObserVale/1
  Constant4/1 -> HWA_CLF_Target_TargetDxConfirm_ObserVale/1
  Constant3/1 -> HWA_CLF_Target_TrgMovDir_ObserVale/1
  Constant1/1 -> HWA_CLF_Target_FusionType_ObserVale/1
  Constant2/1 -> HWA_CLF_Target_2_TargeConfirm/1

== system PubIfDecisionTOS_MDL/TOS_20201112/TOS_2012080320/TOS/LC_LCKie_ELK/TOS_HWA/CurrentLane/HWA_CurrentLane_Target/HWA_CLF_Target_2/HWA_CLF_Target ==
  HWA_CLF_Target_2_Index : Inport
  Object_Fus_Type : Inport  Port=2
  object_MovingState : Inport  Port=3
  PP_ObjMovingDirSignalProcessing : Inport  Port=4
  Object_HeadingAngle : Inport  Port=5
  Object_DX : Inport  Port=6
  TOS_TLJ_SameLaneConfirm_Flag : Inport  Port=7
  Object_Type : Inport  Port=8
  Object_ObstacleProb : Inport  Port=9
  Object_DY : Inport  Port=10
  PP_ObjFusType_FC_FR_Confirm : Inport  Port=11
  PP_ObjFusType_FR_Confirm : Inport  Port=12
  PP_ObjFusType_FC_Confirm : Inport  Port=13
  Object_VX : Inport  Port=14
  Object_VY : Inport  Port=15
  VIE_EgoVelocity : Inport  Port=16
  SteerWheelAng : Inport  Port=17
  PIL_OverlapRatio : Inport  Port=18
  HWA_CLF_Target_ID_K1 : Inport  Port=19
  HWA_CLF_Target_Target_ID_K2 : Inport  Port=20
  HWA_CLF_Target_Target_MovState_K1 : Inport  Port=21
  HWA_CLF_Target_Target_MovState_K2 : Inport  Port=22
  ObjectID : Inport  Port=23
  LM_LR_Line04_dDisStart : Inport  Port=24
  LM_LR_Line04_dDisEnd : Inport  Port=25
  LM_LR_Line05_dDisStart : Inport  Port=26
  LM_LR_Line05_dDisEnd : Inport  Port=27
  LM_LR_Line06_dDisStart : Inport  Port=28
  LM_LR_Line06_dDisEnd : Inport  Port=29
  LM_LR_Line04_pC2 : Inport  Port=30
  LM_LR_Line05_pC2 : Inport  Port=31
  LM_LR_Line06_pC2 : Inport  Port=32
  LM_LR_Line04_fCamValid : Inport  Port=33
  LM_LR_Line05_fCamValid : Inport  Port=34
  LM_LR_Line06_fCamValid : Inport  Port=35
  LM_LR_Line04_pC0 : Inport  Port=36
  LM_RL_Line04_pC0 : Inport  Port=37
  Action Port : ActionPort  ActionPortLabel=else
  HWA_CLF_Target : Subsystem
  Selector{1..16} (16 alike) : Selector  InputPortWidth=80  IndexOptions=Index vector (port)  Indices=[1 3]  OutputSizes=1
  HWA_CLF_Target_2_TargeConfirm : Outport
  HWA_CLF_Target_FusionType_ObserVale : Outport  Port=2
  HWA_CLF_Target_TrgMovDir_ObserVale : Outport  Port=3
  HWA_CLF_Target_TargetDxConfirm_ObserVale : Outport  Port=4
  HWA_CLF_Target_ObjType_ObserVale : Outport  Port=5
  HWA_CLF_Target_ObstacleProb_ObserVale : Outport  Port=6
  HWA_CLF_Target_DyConfirm_ObserVale : Outport  Port=7
  HWA_CLF_Target_TrgMovDirFlag_1_ObserVale : Outport  Port=8
  HWA_CLF_Target_TrgMovDirFlag_2_ObserVale : Outport  Port=9
  HWA_CLF_Target_TrgMovDirFlag_3_ObserVale : Outport  Port=10
  HWA_CLF_Target_TrgMovDirFlag_4_ObserVale : Outport  Port=11
  HWA_CLF_Target_TrgMovDirFlag_5_ObserVale : Outport  Port=12
  HWA_CLF_Target_TrgMovDirFlag_6_ObserVale : Outport  Port=13
  HWA_CLF_Target_DyConfirm_1_ObserVale : Outport  Port=14
  HWA_CLF_Target_DyConfirm_2_ObserVale : Outport  Port=15
  HWA_CLF_Target_DyConfirm_3_ObserVale : Outport  Port=16
  HWA_CLF_Target_DyConfirm_4_OverlapRatio_ObserVale : Outport  Port=17
  HWA_CLF_Target_DyConfirm_5_OverlapConfirm_ObserVale : Outport  Port=18
  HWA_CLF_Target_DyConfirm_ALL_6_ObserVale : Outport  Port=19
  wires:
  Object_Fus_Type/1 -> Selector1/1
  object_MovingState/1 -> Selector13/1
  PP_ObjMovingDirSignalProcessing/1 -> Selector12/1
  Object_HeadingAngle/1 -> Selector16/1
  Object_DX/1 -> Selector15/1
  TOS_TLJ_SameLaneConfirm_Flag/1 -> Selector14/1
  Object_Type/1 -> Selector11/1
  Object_ObstacleProb/1 -> Selector10/1
  Object_DY/1 -> Selector9/1
  PP_ObjFusType_FC_FR_Confirm/1 -> Selector8/1
  PP_ObjFusType_FR_Confirm/1 -> Selector7/1
  PP_ObjFusType_FC_Confirm/1 -> Selector6/1
  Object_VX/1 -> Selector5/1
  Object_VY/1 -> Selector2/1
  VIE_EgoVelocity/1 -> HWA_CLF_Target/15(VIE_EgoVelocity)
  SteerWheelAng/1 -> HWA_CLF_Target/16(SteerWheelAng)
  PIL_OverlapRatio/1 -> Selector4/1
  HWA_CLF_Target_ID_K1/1 -> HWA_CLF_Target/18(HWA_CLF_Target_ID_K1)
  HWA_CLF_Target_Target_ID_K2/1 -> HWA_CLF_Target/19(HWA_CLF_Target_ID_K2)
  HWA_CLF_Target_Target_MovState_K1/1 -> HWA_CLF_Target/20(HWA_CLF_Target_MovState_K1)
  HWA_CLF_Target_Target_MovState_K2/1 -> HWA_CLF_Target/21(HWA_CLF_Target_MovState_K2)
  ObjectID/1 -> Selector3/1
  Selector1/1 -> HWA_CLF_Target/1(Object_Fus_Type)
  Selector13/1 -> HWA_CLF_Target/2(object_MovingState)
  Selector12/1 -> HWA_CLF_Target/3(PP_ObjMovingDirSignalProcessing)
  Selector16/1 -> HWA_CLF_Target/4(Object_HeadingAngle)
  Selector15/1 -> HWA_CLF_Target/5(Object_DX)
  Selector14/1 -> HWA_CLF_Target/6(TOS_TLJ_SameLaneConfirm_Flag)
  Selector11/1 -> HWA_CLF_Target/7(Object_Type)
  Selector10/1 -> HWA_CLF_Target/8(Object_ObstacleProb)
  Selector9/1 -> HWA_CLF_Target/9(Object_DY)
  Selector8/1 -> HWA_CLF_Target/10(PP_ObjFusType_FC_FR_Confirm)
  Selector7/1 -> HWA_CLF_Target/11(PP_ObjFusType_FR_Confirm)
  Selector6/1 -> HWA_CLF_Target/12(PP_ObjFusType_FC_Confirm)
  Selector5/1 -> HWA_CLF_Target/13(Object_VX)
  Selector2/1 -> HWA_CLF_Target/14(Object_VY)
  Selector4/1 -> HWA_CLF_Target/17(PIL_OverlapRatio)
  Selector3/1 -> HWA_CLF_Target/22(ObjectID)
  HWA_CLF_Target_2_Index/1 -> Selector1/2, Selector13/2, Selector12/2, Selector15/2, Selector3/2, Selector4/2, Selector2/2, Selector5/2, Selector6/2, Selector7/2, Selector8/2, Selector9/2, Selector10/2, Selector11/2, Selector14/2, Selector16/2
  LM_LR_Line06_pC2/1 -> HWA_CLF_Target/31(LM_LR_Line06_pC2)
  LM_LR_Line04_dDisStart/1 -> HWA_CLF_Target/23(LM_LR_Line04_dDisStart)
  LM_LR_Line04_dDisEnd/1 -> HWA_CLF_Target/24(LM_LR_Line04_dDisEnd)
  LM_LR_Line05_dDisStart/1 -> HWA_CLF_Target/25(LM_LR_Line05_dDisStart)
  LM_LR_Line05_dDisEnd/1 -> HWA_CLF_Target/26(LM_LR_Line05_dDisEnd)
  LM_LR_Line06_dDisStart/1 -> HWA_CLF_Target/27(LM_LR_Line06_dDisStart)
  LM_LR_Line06_dDisEnd/1 -> HWA_CLF_Target/28(LM_LR_Line06_dDisEnd)
  LM_LR_Line04_pC2/1 -> HWA_CLF_Target/29(LM_LR_Line04_pC2)
  LM_LR_Line05_pC2/1 -> HWA_CLF_Target/30(LM_LR_Line05_pC2)
  LM_LR_Line06_fCamValid/1 -> HWA_CLF_Target/34(LM_LR_Line06_fCamValid)
  LM_LR_Line04_fCamValid/1 -> HWA_CLF_Target/32(LM_LR_Line04_fCamValid)
  LM_LR_Line05_fCamValid/1 -> HWA_CLF_Target/33(LM_LR_Line05_fCamValid)
  HWA_CLF_Target/6(TOS_ObstacleProb_ObserVale) -> HWA_CLF_Target_ObstacleProb_ObserVale/1
  HWA_CLF_Target/7(TOS_DyConfirm_ObserVale) -> HWA_CLF_Target_DyConfirm_ObserVale/1
  HWA_CLF_Target/5(TOS_ObjType_ObserVale) -> HWA_CLF_Target_ObjType_ObserVale/1
  HWA_CLF_Target/8(TOS_TrgMovDirFlag_1_ObserVale) -> HWA_CLF_Target_TrgMovDirFlag_1_ObserVale/1
  HWA_CLF_Target/4(TOS_TargetDxConfirm_ObserVale) -> HWA_CLF_Target_TargetDxConfirm_ObserVale/1
  HWA_CLF_Target/9(TOS_TrgMovDirFlag_2_ObserVale) -> HWA_CLF_Target_TrgMovDirFlag_2_ObserVale/1
  HWA_CLF_Target/3(TOS_TrgMovDir_ObserVale) -> HWA_CLF_Target_TrgMovDir_ObserVale/1
  HWA_CLF_Target/10(TOS_TrgMovDirFlag_3_ObserVale) -> HWA_CLF_Target_TrgMovDirFlag_3_ObserVale/1
  HWA_CLF_Target/2(TOS_FusionType_ObserVale) -> HWA_CLF_Target_FusionType_ObserVale/1
  HWA_CLF_Target/11(TOS_TrgMovDirFlag_4_ObserVale) -> HWA_CLF_Target_TrgMovDirFlag_4_ObserVale/1
  HWA_CLF_Target/1(HWA_CLF_TargeConfirm) -> HWA_CLF_Target_2_TargeConfirm/1
  HWA_CLF_Target/12(TOS_TrgMovDirFlag_5_ObserVale) -> HWA_CLF_Target_TrgMovDirFlag_5_ObserVale/1
  HWA_CLF_Target/13(TOS_TrgMovDirFlag_6_ObserVale) -> HWA_CLF_Target_TrgMovDirFlag_6_ObserVale/1
  HWA_CLF_Target/14(TOS_DyConfirm_1_ObserVale) -> HWA_CLF_Target_DyConfirm_1_ObserVale/1
  HWA_CLF_Target/15(TOS_DyConfirm_2_ObserVale) -> HWA_CLF_Target_DyConfirm_2_ObserVale/1
  HWA_CLF_Target/16(TOS_DyConfirm_3_ObserVale) -> HWA_CLF_Target_DyConfirm_3_ObserVale/1
  HWA_CLF_Target/17(TOS_DyConfirm_4_OverlapRatio_ObserVale) -> HWA_CLF_Target_DyConfirm_4_OverlapRatio_ObserVale/1
  HWA_CLF_Target/18(TOS_DyConfirm_5_OverlapConfirm_ObserVale) -> HWA_CLF_Target_DyConfirm_5_OverlapConfirm_ObserVale/1
  HWA_CLF_Target/19(TOS_DyConfirm_ALL_6_ObserVale) -> HWA_CLF_Target_DyConfirm_ALL_6_ObserVale/1
  LM_LR_Line04_pC0/1 -> HWA_CLF_Target/35(LM_LR_Line04_pC0)
  LM_RL_Line04_pC0/1 -> HWA_CLF_Target/36(LM_RL_Line04_pC0)

== system PubIfDecisionTOS_MDL/TOS_20201112/TOS_2012080320/TOS/LC_LCKie_ELK/TOS_HWA/CurrentLane/HWA_CurrentLane_Target/HWA_CLF_Target_2/HWA_CLF_TargetDefault ==
  Action Port : ActionPort  ActionPortLabel=if(u1 ~= 0)
  Constant{1..19} (19 alike) : Constant  Value=0  OutDataTypeStr=boolean
  HWA_CLF_Target_2_TargeConfirm : Outport
  HWA_CLF_Target_FusionType_ObserVale : Outport  Port=2
  HWA_CLF_Target_TrgMovDir_ObserVale : Outport  Port=3
  HWA_CLF_Target_TargetDxConfirm_ObserVale : Outport  Port=4
  HWA_CLF_Target_ObjType_ObserVale : Outport  Port=5
  HWA_CLF_Target_ObstacleProb_ObserVale : Outport  Port=6
  HWA_CLF_Target_DyConfirm_ObserVale : Outport  Port=7
  HWA_CLF_Target_TrgMovDirFlag_1_ObserVale : Outport  Port=8
  HWA_CLF_Target_TrgMovDirFlag_2_ObserVale : Outport  Port=9
  HWA_CLF_Target_TrgMovDirFlag_3_ObserVale : Outport  Port=10
  HWA_CLF_Target_TrgMovDirFlag_4_ObserVale : Outport  Port=11
  HWA_CLF_Target_TrgMovDirFlag_5_ObserVale : Outport  Port=12
  HWA_CLF_Target_TrgMovDirFlag_6_ObserVale : Outport  Port=13
  HWA_CLF_Target_DyConfirm_1_ObserVale : Outport  Port=14
  HWA_CLF_Target_DyConfirm_2_ObserVale : Outport  Port=15
  HWA_CLF_Target_DyConfirm_3_ObserVale : Outport  Port=16
  HWA_CLF_Target_DyConfirm_4_OverlapRatio_ObserVale : Outport  Port=17
  HWA_CLF_Target_DyConfirm_5_OverlapConfirm_ObserVale : Outport  Port=18
  HWA_CLF_Target_DyConfirm_ALL_6_ObserVale : Outport  Port=19
  wires:
  Constant2/1 -> HWA_CLF_Target_2_TargeConfirm/1
  Constant1/1 -> HWA_CLF_Target_FusionType_ObserVale/1
  Constant3/1 -> HWA_CLF_Target_TrgMovDir_ObserVale/1
  Constant4/1 -> HWA_CLF_Target_TargetDxConfirm_ObserVale/1
  Constant5/1 -> HWA_CLF_Target_ObjType_ObserVale/1
  Constant6/1 -> HWA_CLF_Target_ObstacleProb_ObserVale/1
  Constant7/1 -> HWA_CLF_Target_DyConfirm_ObserVale/1
  Constant8/1 -> HWA_CLF_Target_TrgMovDirFlag_1_ObserVale/1
  Constant9/1 -> HWA_CLF_Target_TrgMovDirFlag_2_ObserVale/1
  Constant10/1 -> HWA_CLF_Target_TrgMovDirFlag_3_ObserVale/1
  Constant11/1 -> HWA_CLF_Target_TrgMovDirFlag_4_ObserVale/1
  Constant12/1 -> HWA_CLF_Target_TrgMovDirFlag_5_ObserVale/1
  Constant13/1 -> HWA_CLF_Target_TrgMovDirFlag_6_ObserVale/1
  Constant14/1 -> HWA_CLF_Target_DyConfirm_2_ObserVale/1
  Constant15/1 -> HWA_CLF_Target_DyConfirm_3_ObserVale/1
  Constant16/1 -> HWA_CLF_Target_DyConfirm_4_OverlapRatio_ObserVale/1
  Constant17/1 -> HWA_CLF_Target_DyConfirm_1_ObserVale/1
  Constant18/1 -> HWA_CLF_Target_DyConfirm_5_OverlapConfirm_ObserVale/1
  Constant19/1 -> HWA_CLF_Target_DyConfirm_ALL_6_ObserVale/1

== system PubIfDecisionTOS_MDL/TOS_20201112/TOS_2012080320/TOS/LC_LCKie_ELK/TOS_HWA/CurrentLane/HWA_CurrentLane_Target/HWA_CLF_Target_3/HWA_CLR_Target ==
  HWA_CurrentLane_ObjIndex : Inport
  PP_ObjMovingDirSignalProcessing : Inport  Port=2
  Object_VX : Inport  Port=3
  Object_VY : Inport  Port=4
  Object_Type : Inport  Port=5
  object_MovingState : Inport  Port=6
  TOS_TLJ_SameLaneConfirm_Flag : Inport  Port=7
  Object_DX : Inport  Port=8
  Object_DY : Inport  Port=9
  Object_Fus_Type : Inport  Port=10
  Object_HeadingAngle : Inport  Port=11
  PP_ObjFusType_FC_FR_Confirm : Inport  Port=12
  PP_ObjFusType_FR_Confirm : Inport  Port=13
  PP_ObjFusType_FC_Confirm : Inport  Port=14
  VIE_EgoVelocity : Inport  Port=15
  Action Port : ActionPort  ActionPortLabel=else
  HWA_CLR_Target : Subsystem
  Selector{,1..12} (13 alike) : Selector  InputPortWidth=80  IndexOptions=Index vector (port)  Indices=[1 3]  OutputSizes=1
  HWA_CLR_Target_3_TargeConfirm : Outport
  HWA_CLR_Target_3_MovState_ObserVale : Outport  Port=2
  HWA_CLR_Target_3_ObjType_ObserVale : Outport  Port=3
  HWA_CLR_Target_3_InCurrentLane_Flag_ObserVale : Outport  Port=4
  HWA_CLR_Target_3_TargetMovingDir_ObserVale : Outport  Port=5
  HWA_CLR_Target_3_DyConfirm_ObserVale : Outport  Port=6
  wires:
  HWA_CLR_Target/5(HWA_CLR_Target_3_TargetMovingDir_ObserVale) -> HWA_CLR_Target_3_TargetMovingDir_ObserVale/1
  HWA_CLR_Target/4(HWA_CLR_Target_3_InCurrentLane_Flag_ObserVale) -> HWA_CLR_Target_3_InCurrentLane_Flag_ObserVale/1
  HWA_CLR_Target/3(HWA_CLR_Target_3_ObjType_ObserVale) -> HWA_CLR_Target_3_ObjType_ObserVale/1
  HWA_CLR_Target/2(HWA_CLR_Target_3_MovState_ObserVale) -> HWA_CLR_Target_3_MovState_ObserVale/1
  HWA_CLR_Target/6(HWA_CLR_Target_3_DyConfirm_ObserVale) -> HWA_CLR_Target_3_DyConfirm_ObserVale/1
  Selector12/1 -> HWA_CLR_Target/9(Object_DY)
  Object_DY/1 -> Selector12/1  "Object_DY"
  HWA_CurrentLane_ObjIndex/1 -> Selector2/2, Selector3/2, Selector4/2, Selector5/2, Selector6/2, Selector7/2, Selector8/2, Selector9/2, Selector10/2, Selector11/2, Selector12/2, Selector1/2, Selector/2  "HWA_CurrentLane_ObjIndex"
  Object_HeadingAngle/1 -> Selector4/1  "Object_HeadingAngle"
  PP_ObjMovingDirSignalProcessing/1 -> Selector3/1  "PP_ObjMovingDirSignalProcessing"
  Object_VX/1 -> Selector/1  "Object_VX"
  Object_VY/1 -> Selector1/1  "Object_VY"
  Object_Type/1 -> Selector5/1  "Object_Type"
  TOS_TLJ_SameLaneConfirm_Flag/1 -> Selector6/1  "TOS_TLJ_SameLaneConfirm_Flag"
  Object_DX/1 -> Selector7/1  "Object_DX"
  Object_Fus_Type/1 -> Selector8/1  "Object_Fus_Type"
  PP_ObjFusType_FC_FR_Confirm/1 -> Selector9/1  "PP_ObjFusType_FC_FR_Confirm"
  PP_ObjFusType_FR_Confirm/1 -> Selector10/1  "PP_ObjFusType_FR_Confirm"
  PP_ObjFusType_FC_Confirm/1 -> Selector11/1  "PP_ObjFusType_FC_Confirm"
  object_MovingState/1 -> Selector2/1  "object_MovingState"
  Selector11/1 -> HWA_CLR_Target/13(PP_ObjFusType_FC_Confirm)
  Selector10/1 -> HWA_CLR_Target/12(PP_ObjFusType_FR_Confirm)
  Selector9/1 -> HWA_CLR_Target/11(PP_ObjFusType_FC_FR_Confirm)
  Selector8/1 -> HWA_CLR_Target/10(Object_Fus_Type)
  Selector7/1 -> HWA_CLR_Target/8(Object_DX)
  Selector6/1 -> HWA_CLR_Target/7(TOS_TLJ_SameLaneConfirm_Flag)
  Selector5/1 -> HWA_CLR_Target/6(Object_Type)
  Selector4/1 -> HWA_CLR_Target/5(Object_HeadingAngle)
  Selector3/1 -> HWA_CLR_Target/4(PP_ObjMovingDirSignalProcessing)
  Selector2/1 -> HWA_CLR_Target/3(object_MovingState)
  Selector1/1 -> HWA_CLR_Target/2(Object_VY)
  Selector/1 -> HWA_CLR_Target/1(Object_VX)
  VIE_EgoVelocity/1 -> HWA_CLR_Target/14(VIE_EgoVelocity)  "VIE_EgoVelocity"
  HWA_CLR_Target/1(HWA_CLR_Target_3_TargeConfirm) -> HWA_CLR_Target_3_TargeConfirm/1
